simulink model "Lab1_nonadaptive"  (R2022b)
settings: Solver=VariableStepAuto  StartTime=0.0  StopTime=t  MaxStep=0.01  RelTol=1e-3
undefined symbols (not defined in the file): lambda, theta
settings Model: Creator=DuPont  LastModifiedBy=DuPont

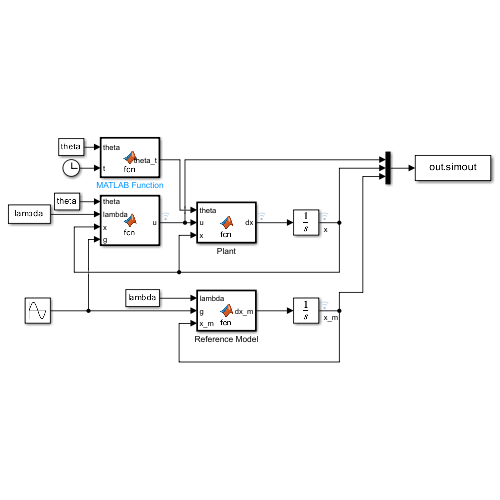
[thumbnail: Simulink's stored preview of the top-level diagram]
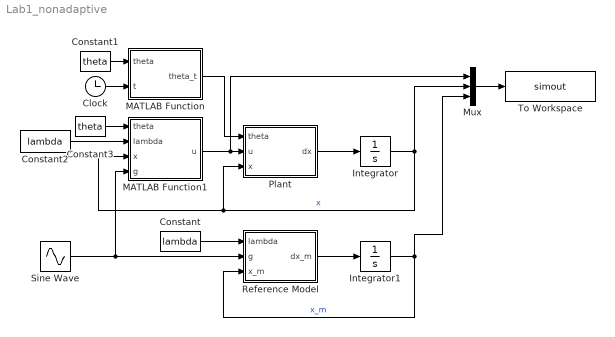
== system Lab1_nonadaptive ==
  Clock : Clock
  Constant : Constant  Value=lambda
  Constant1 : Constant  Value=theta
  Constant2 : Constant  Value=lambda
  Constant3 : Constant  Value=theta
  Integrator : Integrator
  Integrator1 : Integrator
  MATLAB Function : MATLAB Function  TreatAsAtomicUnit=on
  MATLAB Function1 : MATLAB Function  TreatAsAtomicUnit=on
  Mux : Mux  Inputs=3
  Plant : MATLAB Function  TreatAsAtomicUnit=on
  Reference Model : MATLAB Function  TreatAsAtomicUnit=on
  Sine Wave : Sin  Bias=2  Frequency=8  SampleTime=0
  To Workspace : ToWorkspace  VariableName=simout  SaveFormat=Structure With Time  SampleTime=-1
  wires:
  Plant/1(dx) -> Integrator/1
  Reference Model/1(dx_m) -> Integrator1/1
  Constant/1 -> Reference Model/1(lambda)
  Sine Wave/1 -> MATLAB Function1/4(g), Reference Model/2(g)
  Integrator1/1 -> Mux/3, Reference Model/3(x_m)  "x_m"
  Integrator/1 -> Mux/2, Plant/3(x), MATLAB Function1/3(x)  "x"
  MATLAB Function1/1(u) -> Mux/1, Plant/2(u)
  MATLAB Function/1(theta_t) -> Plant/1(theta)
  Constant1/1 -> MATLAB Function/1(theta)
  Clock/1 -> MATLAB Function/2(t)
  Constant2/1 -> MATLAB Function1/2(lambda)
  Constant3/1 -> MATLAB Function1/1(theta)
  Mux/1 -> To Workspace/1

== matlab function Lab1_nonadaptive/Reference Model ==
  data: lambda input; dx_m output; g input; x_m input
function dx_m = fcn(lambda, g, x_m)

dx_m = -lambda*x_m + lambda*g;

== matlab function Lab1_nonadaptive/Plant ==
  data: theta input; u input; x input; dx output
function dx = fcn(theta, u, x)

dx = theta*x + u;

== matlab function Lab1_nonadaptive/MATLAB Function ==
  data: theta input; theta_t output; t input
function theta_t = fcn(theta, t)

if t < 10
    theta_t = theta;
else 
    theta_t = theta*3;
end

== matlab function Lab1_nonadaptive/MATLAB Function1 ==
  data: theta input; u output; lambda input; x input; g input
function u = fcn(theta, lambda, x, g)

u = -theta*x - lambda*x + lambda*g;
